simulink subsystem "sensor_baro"  (R2025b)
settings: Solver=VariableStepAuto  StartTime=0.0  StopTime=10.0  RelTol=1e-3
model mask{samplingrate=100, noise_pres=0.2, bias_pres=0, scale_pres=1, limit_pres=[0, inf]}
  mask prompts: samplingrate "Sampling Rate (Hz)"; noise_pres "Pressure Noise Power"; bias_pres "Pressure Bias"; scale_pres "Pressure Scaling"; limit_pres "Pressure Limit"
libraries: simulink x1, aerolibatmos2 x1
settings Model: Creator=finnb  LastModifiedBy=finnb

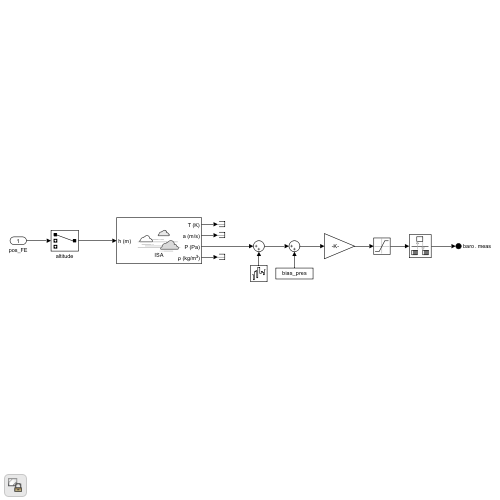
[thumbnail: Simulink's stored preview of the top-level diagram]
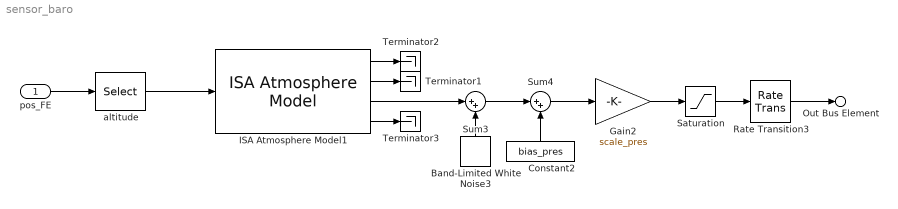
== system sensor_baro ==
  pos_FE : Inport
  Band-Limited White Noise3 : simulink/Sources/Band-Limited White Noise  Cov=noise_pres  Ts=samplingrate  seed=[5781]
  Constant2 : Constant  Value=bias_pres
  Gain2 : Gain  Gain=scale_pres
  ISA Atmosphere Model1 : aerolibatmos2/ISA Atmosphere Model  useExtended=on  action=Warning  custom=off  viscosityOut=off  g=9.80665  gamma=1.4  R=287.0531  L=0.0065  h_trop=11000  h_strat=20000  rho0=1.225  P0=101325  T0=288.15  h0=0  S=110.4  Tref=273.15  muref=1.716e-5
  Rate Transition3 : RateTransition  OutPortSampleTime=samplingrate
  Saturation : Saturate  UpperLimit=limit_pres(2)  LowerLimit=limit_pres(1)
  Sum3 : Sum  Inputs=|++
  Sum4 : Sum  Inputs=|++
  Terminator1 : Terminator
  Terminator2 : Terminator
  Terminator3 : Terminator
  altitude : Selector  InputPortWidth=3  IndexOptions=Index vector (dialog)  Indices=[1]  OutputSizes=1
  Out Bus Element : Outport  PortName=baro  Element=meas
  wires:
  Sum3/1 -> Sum4/1
  ISA Atmosphere Model1/3 -> Sum3/1
  Band-Limited White Noise3/1 -> Sum3/2
  pos_FE/1 -> altitude/1
  altitude/1 -> ISA Atmosphere Model1/1
  ISA Atmosphere Model1/2 -> Terminator1/1
  ISA Atmosphere Model1/4 -> Terminator3/1
  Sum4/1 -> Gain2/1
  Constant2/1 -> Sum4/2
  Gain2/1 -> Saturation/1
  Saturation/1 -> Rate Transition3/1
  Rate Transition3/1 -> Out Bus Element/1
  ISA Atmosphere Model1/1 -> Terminator2/1
